simulink model "untitled"  (R2018a)
settings: Solver=VariableStepAuto  StartTime=0.0  StopTime=10.0  RelTol=1e-3
settings Model: Creator=Muhammad Naufal  LastModifiedBy=Muhammad Naufal

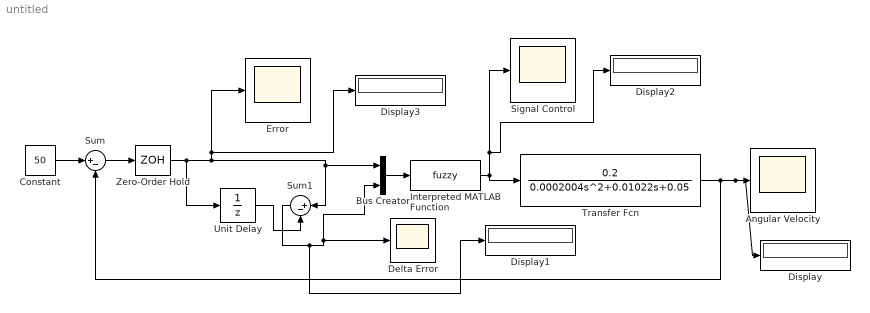
== system untitled ==
  Angular Velocity : Scope
  Bus Creator : BusCreator  Inputs=2
  Constant : Constant  Value=50
  Delta Error : Scope
  Display{,1..3} (4 alike) : Display
  Error : Scope
  Interpreted MATLAB Function : MATLABFcn  MATLABFcn=fuzzy
  Signal Control : Scope
  Sum : Sum  Inputs=|+-
  Sum1 : Sum  Inputs=|+-
  Transfer Fcn : TransferFcn  Numerator=[0.2]  Denominator=[0.0002004 0.01022 0.05]
  Unit Delay : UnitDelay  SampleTime=0.001
  Zero-Order Hold : ZeroOrderHold  SampleTime=0.001
  wires:
  Constant/1 -> Sum/1
  Sum/1 -> Zero-Order Hold/1
  Zero-Order Hold/1 -> Display3/1, Error/1, Bus Creator/1, Sum1/1, Unit Delay/1
  Unit Delay/1 -> Sum1/2
  Sum1/1 -> Bus Creator/2, Delta Error/1, Display1/1
  Bus Creator/1 -> Interpreted MATLAB Function/1
  Interpreted MATLAB Function/1 -> Display2/1, Signal Control/1, Transfer Fcn/1
  Transfer Fcn/1 -> Display/1, Angular Velocity/1, Sum/2
